simulink model "Phase_Estimation_tunable"  (Simulink 8.7)
settings: Solver=ode3  StartTime=0.0  StopTime=t(end)  FixedStep=1/60  RelTol=1e-3
values from neighbouring files (symbols this model uses):
  Data = [0:1/60:400]'    [Adaptive_notch_filter.m]    (also in Evolutionary_Strategy_ANF_mutation.m)
  gamma_d = 0.0324    [Adaptive_notch_filter.m]    (also in Evolutionary_Strategy_ANF_mutation.m = mean(Gamma_d))
  gamma_omg = 2.0893*10^(-10)    (= 2.0893e-10)    [Adaptive_notch_filter.m]    (also in Evolutionary_Strategy_ANF_mutation.m = mean(Gamma_omg))
  x_initial = [0 0 0 0 0 0 0 0 0 0 0 2*pi/24]    [Adaptive_notch_filter.m]    (also in Evolutionary_Strategy_ANF_mutation.m = [0 0 0 0 0 0 0 2*pi/24])
  zeta = 0.0599    [Adaptive_notch_filter.m]    (also in Evolutionary_Strategy_ANF_mutation.m = mean(Zeta))
settings Model: Creator=wangf7  LastModifiedBy=Jiawei Yin
settings OptimizationCC: ExpressionDepthLimit=2147483647
settings DebuggingCC: SolverPrmCheckMsg=warning  StateNameClashWarn=warning
settings ConfigurationSet: Description=SimMechanics 2G

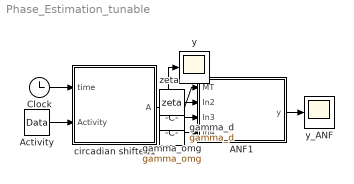
== system Phase_Estimation_tunable ==
  ANF1 : Subsystem
  Activity : Constant  Value=Data
  Clock : Clock
  circadian shifted1 : MATLAB Function  TreatAsAtomicUnit=on
  gamma_d : Constant  Value=gamma_d
  gamma_omg : Constant  Value=gamma_omg
  y : Scope
  y_ANF : Scope
  zeta : Constant  Value=zeta
  wires:
  circadian shifted1/1(A) -> y/1, ANF1/1(MT)
  Activity/1 -> circadian shifted1/2(Activity)
  Clock/1 -> circadian shifted1/1(time)
  ANF1/1(y) -> y_ANF/1
  zeta/1 -> ANF1/2(In2)
  gamma_omg/1 -> ANF1/3(In3)
  gamma_d/1 -> ANF1/4(In4)

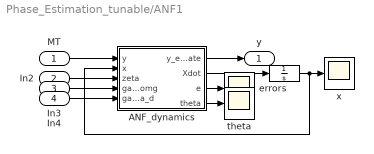
== system Phase_Estimation_tunable/ANF1 ==
  MT : Inport
  In2 : Inport  Port=2
  In3 : Inport  Port=3
  In4 : Inport  Port=4
  ANF_dynamics : MATLAB Function  TreatAsAtomicUnit=on
  error : Scope
  s : Integrator  InitialCondition=x_initial
  theta : Scope
  x : Scope
  y : Outport
  wires:
  MT/1 -> ANF_dynamics/1(y)
  s/1 -> ANF_dynamics/2(x), x/1
  ANF_dynamics/2(Xdot) -> s/1
  ANF_dynamics/1(y_estimate) -> y/1
  ANF_dynamics/3(e) -> error/1
  ANF_dynamics/4(theta) -> theta/1
  In2/1 -> ANF_dynamics/3(zeta)
  In3/1 -> ANF_dynamics/4(gamma_omg)
  In4/1 -> ANF_dynamics/5(gamma_d)

== matlab function circadian shifted1 ==
  data: time input double; Activity input double; A output double
function A = fcn(time,Activity)
%#eml
A=interp1q(Activity(:,1),Activity(:,2),time);

== matlab function ANF1/ANF_dynamics ==
  data: y_estimate output double; y input double; x input double; Xdot output double; e output double; theta output double; zeta input double; gamma_omg input double; gamma_d input double
function [y_estimate,Xdot,e,theta] = fcn(y,x,zeta,gamma_omg,gamma_d)

% zeta = 0.03;
% gamma_omg =  0.00000000001;
% gamma_d = 0.0000001;

x1 = x(1);%1st harmonic
x2 = x(2);%1st harmonic dot
dc = x(3);%dc
omg = x(4);%omega

y_estimate = dc + 2*zeta/omg*x2;
e = y - y_estimate;
if isnan(y)
    e=0;
end

Xdot = zeros(4,1);

Xdot(1,1) = x2;
Xdot(2,1) = omg^2*(e-x1);
Xdot(3,1) = gamma_d*e;
Xdot(4,1) = gamma_omg*(-x1*omg^2)*e;
%y_estimate = dc + 2*zeta/omg*x2;
theta=mod(atan2(x(2),-x(4)*x(1)),2*pi);
